simulink model "FocParamIdentifyModel"  (R2024a)
settings: Solver=FixedStepDiscrete  StartTime=0.0  StopTime=4  FixedStep=0.00005  RelTol=1e-3
values from neighbouring files (symbols this model uses):
  Flux = 0.00084    [FocParamIDFData.mat]
  Ld = 3.62e-05    [FocParamIDFData.mat]
  Lq = 4.24e-05    [FocParamIDFData.mat]
  Pole = 10    [FocParamIDFData.mat]
  Rs = 0.113    [FocParamIDFData.mat]
  Ts = 5e-05    [FocParamIDFData.mat]
undefined symbols (not defined in the file or in its folder): DiscIntNeverNeededParam, magnitude
libraries: slpidlib x4, mcbplantlib x1, autolibpmsmexterior x1
(part 1 of 2)
settings Model: Creator=张先生  LastModifiedBy=张先生
settings OptimizationCC: DefaultParameterBehavior=Inlined  UseDivisionForNetSlopeComputation=on  GainParamInheritBuiltInType=on  UseFloatMulNetSlope=on  InlineInvariantSignals=on  PassReuseOutputArgsAs=Individual arguments  ZeroExternalMemoryAtStartup=off  ZeroInternalMemoryAtStartup=off  NoFixptDivByZeroProtection=on  EfficientFloat2IntCast=on  LifeSpan=1  OptimizeBlockOrder=speed  DifferentSizesBufferReuse=on  EfficientTunableParamExpr=on
settings DebuggingCC: ParameterTunabilityLossMsg=error
settings HardwareCC: ProdBitPerPointer=32  ProdBitPerSizeT=32  ProdBitPerPtrDiffT=32  ProdLargestAtomicInteger=Long  ProdLargestAtomicFloat=Double  ProdWordSize=32  ProdLongLongMode=on  ProdHWDeviceType=ARM Compatible->ARM Cortex-M
settings SFSimCC: MATLABDynamicMemAlloc=off
settings RTWCC: Description=Embedded Coder  SystemTargetFile=ert.tlc  TemplateMakefile=ert_default_tmf  GenerateReport=on  LaunchReport=on
settings CodeAppCC: ForceParamTrailComments=on  IgnoreCustomStorageClasses=off  OperatorAnnotations=on  SimulinkDataObjDesc=on  SFDataObjDesc=on  CustomSymbolStrGlobalVar=rt$N$M  CustomSymbolStrType=$N$M  CustomSymbolStrFcn=$N$M$F  CustomSymbolStrMacro=$N$M  InsertBlockDesc=on
settings ERTTargetCC: TargetLangStandard=C99 (ISO)  CodeReplacementLibrary=ARM Cortex-M  GenerateSampleERTMain=on  IncludeMdlTerminateFcn=off  CombineSignalStateStructs=on  SupportComplex=off  SupportContinuousTime=on  SupportNonInlinedSFcns=on  InlinedParameterPlacement=NonHierarchical  ERTCustomFileTemplate=example_file_process.tlc  ERTFilePackagingFormat=CompactWithDataFile

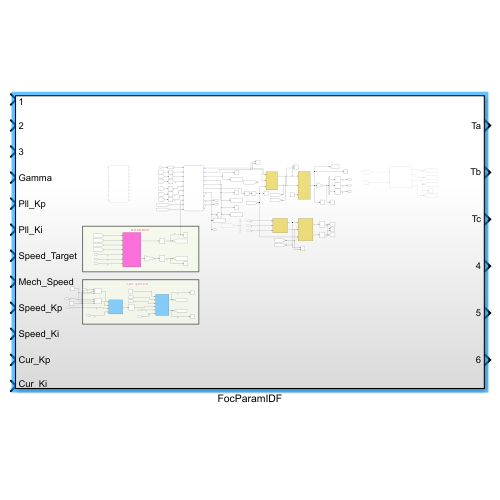
[thumbnail: Simulink's stored preview of the top-level diagram]
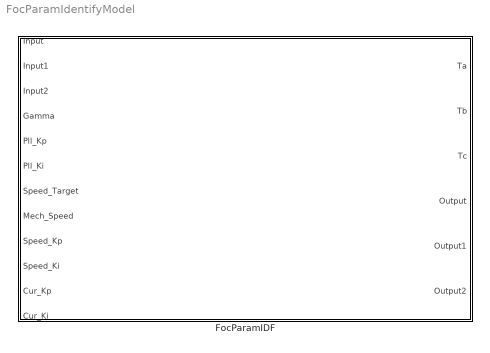
== system FocParamIdentifyModel ==
  FocParamIDF : Subsystem

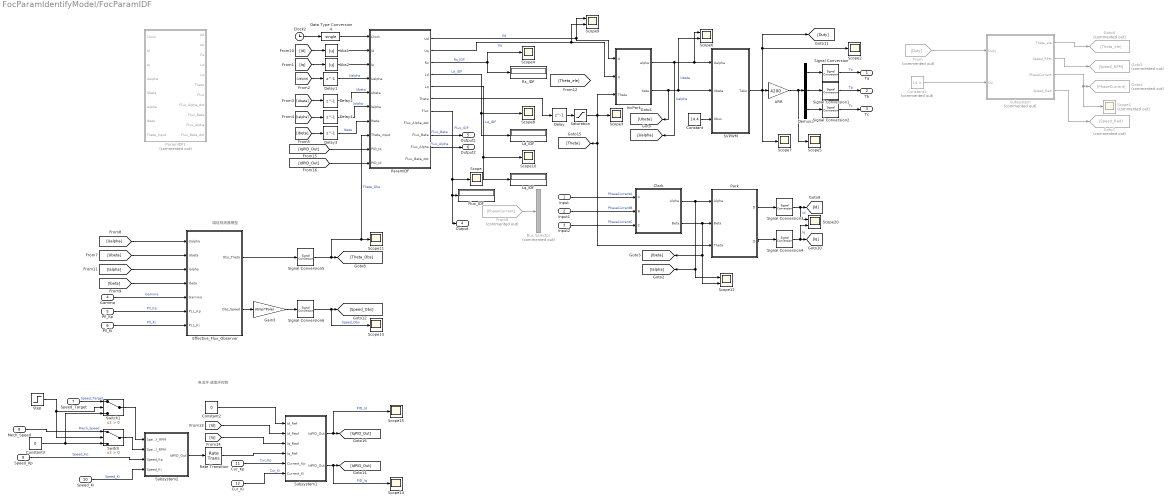
== system FocParamIdentifyModel/FocParamIDF ==
  note: 磁链观测器模型
  note: 电流环 速度环控制
  Input : Inport
  Input1 : Inport  Port=2
  Input2 : Inport  Port=3
  Gamma : Inport  Port=4
  Pll_Kp : Inport  Port=5
  Pll_Ki : Inport  Port=6
  Speed_Target : Inport  Port=7
  Mech_Speed : Inport  Port=8
  Speed_Kp : Inport  Port=9
  Speed_Ki : Inport  Port=10
  Cur_Kp : Inport  Port=11
  Cur_Ki : Inport  Port=12
  ARR : Gain  Gain=4200
  Abs1 : Abs  SaturateOnIntegerOverflow=off
  Abs2 : Abs  SaturateOnIntegerOverflow=off
  Bus Selector : BusSelector  Commented=on  OutputSignals=signal1,signal2,signal3
  Clark : Subsystem  TreatAsAtomicUnit=on
      settings: RTWSystemCode=Inline  RTWFcnNameOpts=Use subsystem name
      mask Display:
      | port_label('input',1,'a','texmode','on');
      | port_label('input',2,'b','texmode','on');
      | port_label('input',3,'c','texmode','on');
      | 
      | port_label('output',1,'\alpha','texmode','on');
      | port_label('output',2,'\beta','texmode','on');
      | 
      | fprintf('Clark');
  Clock2 : Clock
  Constant : Constant  Value=14.4  OutDataTypeStr=single
  Constant1 : Constant  Commented=on  Value=14.4  OutDataTypeStr=single
  Constant2 : Constant  Value=0  OutDataTypeStr=single
  Constant3 : Constant  Value=0  OutDataTypeStr=single
  Data Type Conversion4 : DataTypeConversion  OutDataTypeStr=single  SaturateOnIntegerOverflow=off  RndMeth=Floor
  Delay{,1..4} (5 alike) : Delay  DelayLength=1
  Demux3 : Demux  Outputs=3
  Effective_Flux_Observer : Subsystem
  Flux_IDF : Display
  From : From  Commented=on  GotoTag=Duty
  From6 : From  Commented=on  GotoTag=PhaseCurrent
  Gain3 : Gain  Gain=30/(pi*Pole)
  Goto4 : Goto  Commented=on  GotoTag=PhaseCurrent
  Goto5 : Goto  Commented=on  GotoTag=Speed_RPM
  Goto6 : Goto  Commented=on  GotoTag=Theta_ele
  Goto7 : Goto  Commented=on  GotoTag=Speed_Rad
  InvPark : Subsystem  TreatAsAtomicUnit=on
      settings: RTWFcnNameOpts=Use subsystem name
      mask Display:
      | port_label('input',1,'d','texmode','on');
      | port_label('input',2,'q','texmode','on');
      | port_label('input',3,'\theta','texmode','on');
      | 
      | port_label('output',1,'\alpha','texmode','on');
      | port_label('output',2,'\beta','texmode','on');
      | 
      | fprintf('Inverse\nPark')
  Ld_IDF : Display
  Lq_IDF : Display
  ParamIDF : Stateflow chart  TreatAsAtomicUnit=on
      settings: PortSchema="{\"entries\":[{\"content\":{\"sides\":[{\"content\":{\"connectorIds\":[\"In1\",\"In2\",\"In3\",\"In5\",\"In4\",\"In6\",\"In7\",\"In8\",\"In9\",\"In10\"]},\"type\":\"ConnectorPlacement.EquallySpacedRectSide\",\"uuid\":\"34403095-885b-4e18-8d39-de6823f4686e\"},{\"content\":{\"connectorIds\":[\"Out1\",\"Out3\",\"Out2\",\"Out4\",\"Out5\",\"Out6\",\"Out7\",\"Out8\",\"Out9\",\"Out10\",\"Out11\"],\"side\":\"RIGHT\"},\"type\":\"ConnectorPlacement.EquallySpacedRectSide\",\"uuid\":\"fe9f0ca0-7ade-4e8e-90a3-c920b6aed83b\"},{\"content\":{\"side\":\"TOP\"},\"type\":\"ConnectorPlacement.EquallySpacedRectSide\",\"uuid\":\"529ead30-0d9e-45e7-a0bb-7696b3472c65\"}]},\"type\":\"ConnectorPlacement.EquallySpacedConnector\",\"uuid\":\"00a1794a-fccb-4faf-9016-ac3359af7e1a\"}],\"packageUris\":[\"http://schema.mathworks.com/mf0/Connector/R2020b\"],\"version\":\"1.0\"}"
  ParamIDF1 : Stateflow chart  Commented=on  TreatAsAtomicUnit=on
      settings: PortSchema="{\"entries\":[{\"content\":{\"sides\":[{\"content\":{\"connectorIds\":[\"In1\",\"In2\",\"In3\",\"In5\",\"In4\",\"In6\",\"In7\",\"In8\"]},\"type\":\"ConnectorPlacement.EquallySpacedRectSide\",\"uuid\":\"34403095-885b-4e18-8d39-de6823f4686e\"},{\"content\":{\"connectorIds\":[\"Out1\",\"Out3\",\"Out2\",\"Out4\",\"Out5\",\"Out6\",\"Out7\",\"Out8\",\"Out9\",\"Out10\",\"Out11\"],\"side\":\"RIGHT\"},\"type\":\"ConnectorPlacement.EquallySpacedRectSide\",\"uuid\":\"fe9f0ca0-7ade-4e8e-90a3-c920b6aed83b\"},{\"content\":{\"side\":\"TOP\"},\"type\":\"ConnectorPlacement.EquallySpacedRectSide\",\"uuid\":\"529ead30-0d9e-45e7-a0bb-7696b3472c65\"}]},\"type\":\"ConnectorPlacement.EquallySpacedConnector\",\"uuid\":\"00a1794a-fccb-4faf-9016-ac3359af7e1a\"}],\"packageUris\":[\"http://schema.mathworks.com/mf0/Connector/R2020b\"],\"version\":\"1.0\"}"
  Park : Subsystem  TreatAsAtomicUnit=on
      settings: RTWFcnNameOpts=Use subsystem name
      mask Display:
      | port_label('input',1,'\alpha','texmode','on');
      | port_label('input',2, '\beta','texmode','on');
      | port_label('input',3, '\theta','texmode','on');
      | 
      | port_label('output',1,'d','texmode','on');
      | port_label('output',2,'q','texmode','on');
      | fprintf('Park');
  Rate Transition : RateTransition
  Rs_IDF : Display
  SVPWM : Subsystem  TreatAsAtomicUnit=on
  Saturation : Saturate  UpperLimit=2*pi-0.001  LowerLimit=-2*pi + 0.001
  Scope{,2..5,7..8,10..11,13..15} (12 alike) : Scope
  Scope1 : Scope  Commented=on
  Scope{6,9,12,20} (4 alike) : Scope  NumInputPorts=2
  Signal Conversion{,1..6} (7 alike) : SignalConversion  OverrideOpt=off
  Step : Step  Time=15  OutDataTypeStr=single  SampleTime=0
  Subsystem : Subsystem  Commented=on
  Subsystem1 : Subsystem
  Subsystem2 : Subsystem
  Switch : Switch  Criteria=u2 > Threshold  SaturateOnIntegerOverflow=off  InputSameDT=off
  Switch1 : Switch  Criteria=u2 > Threshold  SaturateOnIntegerOverflow=off  InputSameDT=off
  Ta : Outport
  Tb : Outport  Port=2
  Tc : Outport  Port=3
  Output : Outport  Port=4
  Output1 : Outport  Port=5
  Output2 : Outport  Port=6
  wires:
  Clark/2(Beta) -> Scope12/2, [Ibeta], Park/2(Beta)
  InvPark/1(alpha) -> Scope6/1, SVPWM/1(Ualpha), [Ualpha]  "Ualpha"
  InvPark/2(beta) -> Scope6/2, SVPWM/2(Ubeta), [Ubeta]  "Ubeta"
  Saturation/1 -> InvPark/3(Theta), Scope3/1, [Theta], Park/3(Theta)
  SVPWM/1(Tabc) -> Scope2/1, [Duty], ARR/1, Scope7/1
  ARR/1 -> Scope5/1, Demux3/1
  Park/1(D) -> Signal Conversion3/1
  Signal Conversion4/1 -> Scope20/2, [Iq]  "Iq"
  Signal Conversion2/1 -> Tc/1  "Tc"
  Signal Conversion3/1 -> Scope20/1, [Id]  "Id"
  Signal Conversion/1 -> Ta/1  "Ta"
  Demux3/2 -> Signal Conversion1/1
  Demux3/1 -> Signal Conversion/1
  Park/2(Q) -> Signal Conversion4/1
  Demux3/3 -> Signal Conversion2/1
  Clark/1(Alpha) -> Scope12/1, [Ialpha], Park/1(Alpha)
  Signal Conversion1/1 -> Tb/1  "Tb"
  Constant/1 -> SVPWM/3(Ubus)
  From/1 -> Subsystem/1(Duty)
  Constant1/1 -> Subsystem/2(DC)
  Subsystem/1(Theta_ele) -> Goto6/1
  Subsystem/2(Speed_RPM) -> Goto5/1
  Subsystem/3(PhaseCurrent) -> Scope1/1, Goto4/1
  From6/1 -> Bus Selector/1
  Clock2/1 -> Data Type Conversion4/1
  Data Type Conversion4/1 -> ParamIDF/1(Clock)
  ParamIDF/1(Ud) -> Scope9/1, InvPark/1(d)  "Ud"
  [Id] -> Abs1/1
  Abs1/1 -> ParamIDF/2(Id)
  ParamIDF/4(Ld) -> Scope8/1, Ld_IDF/1  "Ld_IDF"
  ParamIDF/5(Lq) -> Scope10/1, Lq_IDF/1  "Lq_IDF"
  ParamIDF/2(Rs) -> Scope4/1, Rs_IDF/1  "Rs_IDF"
  ParamIDF/3(Uq) -> Scope9/2, InvPark/2(q)  "Uq"
  [Iq] -> Abs2/1
  Abs2/1 -> ParamIDF/3(Iq)
  ParamIDF/6(Theta) -> Delay/1
  [Ualpha] -> Delay1/1
  [Ubeta] -> Delay2/1
  [Ialpha] -> Delay4/1
  [Ibeta] -> Delay3/1
  Delay1/1 -> ParamIDF/5(Ualpha)  "Ualpha"
  Delay2/1 -> ParamIDF/4(Ubeta)  "Ubeta"
  Delay3/1 -> ParamIDF/7(Ibeta)  "Ibeta"
  Delay4/1 -> ParamIDF/6(Ialpha)  "Ialpha"
  ParamIDF/7(Flux) -> Flux_IDF/1, Output/1, Scope/1  "Flux_IDF"
  Delay/1 -> Saturation/1
  Subsystem/4(Speed_Rad) -> Goto7/1
  Input/1 -> Clark/1(A)  "PhaseCurrentA"
  Input1/1 -> Clark/2(B)  "PhaseCurrentB"
  Input2/1 -> Clark/3(C)  "PhaseCurrentC"
  ParamIDF/9(Flux_Beta) -> Output1/1  "Flux_Beta"
  ParamIDF/10(Flux_Alpha) -> Output2/1  "Flux_Alpha"
  Effective_Flux_Observer/2(Obs_Speed) -> Gain3/1
  Signal Conversion5/1 -> [Theta_Obs], Scope11/1, ParamIDF/8(Theta_Input)  "Theta_Obs"
  Gain3/1 -> Signal Conversion6/1
  Pll_Ki/1 -> Effective_Flux_Observer/7(PLL_Ki)  "Pll_Ki"
  Signal Conversion6/1 -> Scope13/1, [Speed_Obs]  "Speed_Obs"
  Pll_Kp/1 -> Effective_Flux_Observer/6(PLL_Kp)  "Pll_Kp"
  Gamma/1 -> Effective_Flux_Observer/5(Gamma)  "Gamma"
  Effective_Flux_Observer/1(Obs_Theta) -> Signal Conversion5/1
  [Id] -> Subsystem1/2(Id_Real)
  Rate Transition/1 -> Subsystem1/4(Iq_Ref)
  Speed_Kp/1 -> Subsystem2/3(Speed_Kp)  "Speed_Kp"
  Cur_Ki/1 -> Subsystem1/6(Current_Ki)  "Cur_Ki"
  Constant2/1 -> Subsystem1/1(Id_Ref)
  Speed_Ki/1 -> Subsystem2/4(Speed_Ki)  "Speed_Ki"
  Subsystem1/1(IqPID_Out) -> Scope15/1, [IqPID_Out]  "PID_Id"
  [Iq] -> Subsystem1/3(Iq_Real)
  Subsystem1/2(IdPID_Out) -> Scope14/1, [IdPID_Out]  "PID_Iq"
  Cur_Kp/1 -> Subsystem1/5(Current_Kp)  "Cur_Kp"
  Subsystem2/1(IdPID_Out) -> Rate Transition/1
  [IqPID_Out] -> ParamIDF/9(PID_Iq)
  [IdPID_Out] -> ParamIDF/10(PID_Id)
  [Ualpha] -> Effective_Flux_Observer/1(Ualpha)
  [Ubeta] -> Effective_Flux_Observer/2(Ubeta)
  [Ialpha] -> Effective_Flux_Observer/3(Ialpha)
  [Ibeta] -> Effective_Flux_Observer/4(Ibeta)
  Mech_Speed/1 -> Switch/1  "Mech_Speed"
  Switch/1 -> Subsystem2/2(Speed_Real_RPM)
  Constant3/1 -> Switch1/3, Switch/3
  Step/1 -> Switch1/2, Switch/2
  Speed_Target/1 -> Switch1/1  "Speed_Target"
  Switch1/1 -> Subsystem2/1(Speed_Ref_RPM)

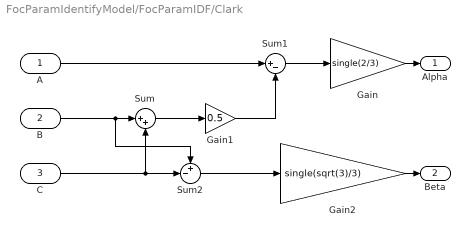
== system FocParamIdentifyModel/FocParamIDF/Clark ==
  A : Inport  OutDataTypeStr=single
  B : Inport  Port=2  OutDataTypeStr=single
  C : Inport  Port=3  OutDataTypeStr=single
  Gain : Gain  Gain=single(2/3)  OutDataTypeStr=single
  Gain1 : Gain  Gain=0.5  OutDataTypeStr=single
  Gain2 : Gain  Gain=single(sqrt(3)/3)  OutDataTypeStr=single
  Sum : Sum  Inputs=|++  OutDataTypeStr=single
  Sum1 : Sum  Inputs=|+-  OutDataTypeStr=single
  Sum2 : Sum  Inputs=+-|  OutDataTypeStr=single
  Alpha : Outport  OutDataTypeStr=single
  Beta : Outport  Port=2  OutDataTypeStr=single
  wires:
  Sum/1 -> Gain1/1
  Gain2/1 -> Beta/1
  B/1 -> Sum2/1, Sum/1
  Gain1/1 -> Sum1/2
  Gain/1 -> Alpha/1
  Sum2/1 -> Gain2/1
  C/1 -> Sum2/2, Sum/2
  A/1 -> Sum1/1
  Sum1/1 -> Gain/1

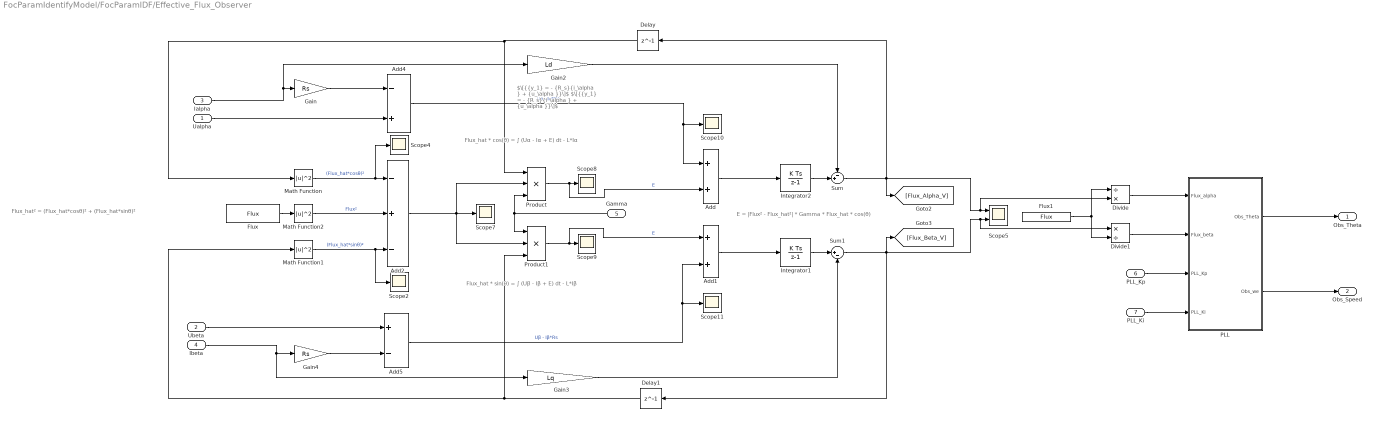
== system FocParamIdentifyModel/FocParamIDF/Effective_Flux_Observer ==
  note: Flux_hat² = (Flux_hat*cosθ)² + (Flux_hat*sinθ)²
  note: E = |Flux² - Flux_hat²| * Gamma * Flux_hat * cos(θ)
  note: Flux_hat * cos(θ) = ∫ (Uα - Iα + E) dt - L*Iα
  note: $\[{{y_1} = - {R_s}{i_\alpha } + {u_\alpha }}\]$ $\[{{y_1} = - {R_s}{i_\alpha } + {u_\alpha }}\]$
  note: Flux_hat * sin(θ) = ∫ (Uβ - Iβ + E) dt - L*Iβ
  Ualpha : Inport  OutDataTypeStr=single
  Ubeta : Inport  Port=2  OutDataTypeStr=single
  Ialpha : Inport  Port=3  OutDataTypeStr=single
  Ibeta : Inport  Port=4  OutDataTypeStr=single
  Gamma : Inport  Port=5
  PLL_Kp : Inport  Port=6
  PLL_Ki : Inport  Port=7
  Add : Sum  OutDataTypeStr=single
  Add1 : Sum  OutDataTypeStr=single
  Add2 : Sum  Inputs=-+-  OutDataTypeStr=single
  Add4 : Sum  Inputs=-+  OutDataTypeStr=single
  Add5 : Sum  Inputs=+-  OutDataTypeStr=single
  Delay : Delay  DelayLength=1
  Delay1 : Delay  DelayLength=1
  Divide : Product  Inputs=/*  OutDataTypeStr=single
  Divide1 : Product  Inputs=*/  OutDataTypeStr=single
  Flux : Constant  Value=Flux  OutDataTypeStr=double
  Flux1 : Constant  Value=Flux  OutDataTypeStr=double
  Gain : Gain  Gain=Rs  OutDataTypeStr=single
  Gain2 : Gain  Gain=Ld  OutDataTypeStr=single
  Gain3 : Gain  Gain=Lq  OutDataTypeStr=single
  Gain4 : Gain  Gain=Rs  OutDataTypeStr=single
  Integrator1 : DiscreteIntegrator  SampleTime=-1  OutDataTypeStr=single  ICPrevOutput=DiscIntNeverNeededParam  ICPrevScaledInput=DiscIntNeverNeededParam  mask(DiscretizedDiscreteIntegrator){}
      mask init:
      | %zoh
  Integrator2 : DiscreteIntegrator  SampleTime=-1  OutDataTypeStr=single  ICPrevOutput=DiscIntNeverNeededParam  ICPrevScaledInput=DiscIntNeverNeededParam  mask(DiscretizedDiscreteIntegrator){}
      mask init:
      | %zoh
  Math Function : Math  Operator=magnitude^2  OutDataTypeStr=single
  Math Function1 : Math  Operator=magnitude^2  OutDataTypeStr=single
  Math Function2 : Math  Operator=magnitude^2  OutDataTypeStr=single
  PLL : Subsystem
  Product : Product  Inputs=3  OutDataTypeStr=single
  Product1 : Product  Inputs=3  OutDataTypeStr=single
  Scope{2,4,7..11} (7 alike) : Scope
  Scope5 : Scope  NumInputPorts=2
  Sum : Sum  Inputs=-+|  OutDataTypeStr=single
  Sum1 : Sum  Inputs=|+-  OutDataTypeStr=single
  Obs_Theta : Outport
  Obs_Speed : Outport  Port=2
  wires:
  Gain2/1 -> Sum/1
  Gamma/1 -> Product1/1, Product/3
  Add5/1 -> Add1/2, Scope11/1  "Uβ - Iβ*Rs"
  Gain3/1 -> Sum1/2
  Integrator2/1 -> Sum/2
  Ialpha/1 -> Gain2/1, Gain/1
  Sum/1 -> [Flux_Alpha_V], Delay/1, Divide/2, Scope5/1
  Add4/1 -> Add/1, Scope10/1  "Uα - Iα*Rs"
  Add2/1 -> Scope7/1, Product1/2, Product/2
  Integrator1/1 -> Sum1/1
  Ibeta/1 -> Gain3/1, Gain4/1
  Sum1/1 -> Divide1/1, Scope5/2, [Flux_Beta_V], Delay1/1
  PLL/1(Obs_Theta) -> Obs_Theta/1
  Math Function1/1 -> Scope2/1, Add2/3  "(Flux_hat*sinθ)²"
  Math Function/1 -> Scope4/1, Add2/1  "(Flux_hat*cosθ)²"
  Product/1 -> Add/2, Scope8/1  "E"
  Product1/1 -> Add1/1, Scope9/1  "E"
  Flux/1 -> Math Function2/1
  Math Function2/1 -> Add2/2  "Flux²"
  Ubeta/1 -> Add5/1
  Gain4/1 -> Add5/2
  PLL/2(Obs_we) -> Obs_Speed/1
  Ualpha/1 -> Add4/2
  PLL_Kp/1 -> PLL/3(PLL_Kp)
  PLL_Ki/1 -> PLL/4(PLL_Ki)
  Add/1 -> Integrator2/1
  Add1/1 -> Integrator1/1
  Delay/1 -> Product/1, Math Function/1
  Delay1/1 -> Product1/3, Math Function1/1
  Gain/1 -> Add4/1
  Divide/1 -> PLL/1(Flux_alpha)
  Divide1/1 -> PLL/2(Flux_beta)
  Flux1/1 -> Divide1/2, Divide/1

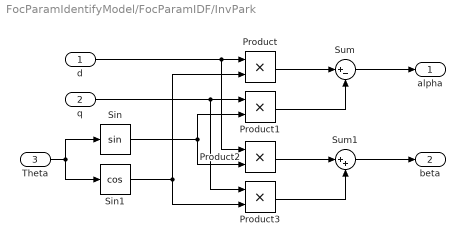
== system FocParamIdentifyModel/FocParamIDF/InvPark ==
  d : Inport  OutDataTypeStr=single
  q : Inport  Port=2  OutDataTypeStr=single
  Theta : Inport  Port=3  OutDataTypeStr=single
  Product{,1..3} (4 alike) : Product  OutDataTypeStr=single
  Sin : Trigonometry  ApproximationMethod=Lookup  TableDataTypeStr=single
  Sin1 : Trigonometry  Operator=cos  ApproximationMethod=Lookup  TableDataTypeStr=single
  Sum : Sum  Inputs=|+-  OutDataTypeStr=single
  Sum1 : Sum  Inputs=|++  OutDataTypeStr=single
  alpha : Outport  OutDataTypeStr=single
  beta : Outport  Port=2  OutDataTypeStr=single
  wires:
  Sum/1 -> alpha/1
  Theta/1 -> Sin1/1, Sin/1
  d/1 -> Product2/1, Product/1
  Sin1/1 -> Product/2, Product3/2
  q/1 -> Product3/1, Product1/1
  Sin/1 -> Product1/2, Product2/2
  Product/1 -> Sum/1
  Product1/1 -> Sum/2
  Product2/1 -> Sum1/1
  Product3/1 -> Sum1/2
  Sum1/1 -> beta/1

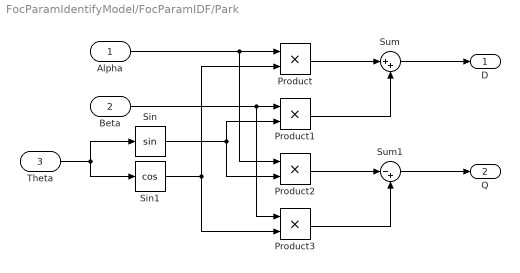
== system FocParamIdentifyModel/FocParamIDF/Park ==
  Alpha : Inport  OutDataTypeStr=single
  Beta : Inport  Port=2  OutDataTypeStr=single
  Theta : Inport  Port=3  OutDataTypeStr=single
  Product{,1..3} (4 alike) : Product  OutDataTypeStr=single
  Sin : Trigonometry  ApproximationMethod=Lookup  TableDataTypeStr=single
  Sin1 : Trigonometry  Operator=cos  ApproximationMethod=Lookup  TableDataTypeStr=single
  Sum : Sum  Inputs=|++  OutDataTypeStr=single
  Sum1 : Sum  Inputs=|-+  OutDataTypeStr=single
  D : Outport  OutDataTypeStr=single
  Q : Outport  Port=2  OutDataTypeStr=single
  wires:
  Beta/1 -> Product3/1, Product1/1
  Alpha/1 -> Product2/1, Product/1
  Theta/1 -> Sin1/1, Sin/1
  Sin1/1 -> Product/2, Product3/2
  Sin/1 -> Product1/2, Product2/2
  Product/1 -> Sum/1
  Product1/1 -> Sum/2
  Sum/1 -> D/1
  Product2/1 -> Sum1/1
  Product3/1 -> Sum1/2
  Sum1/1 -> Q/1

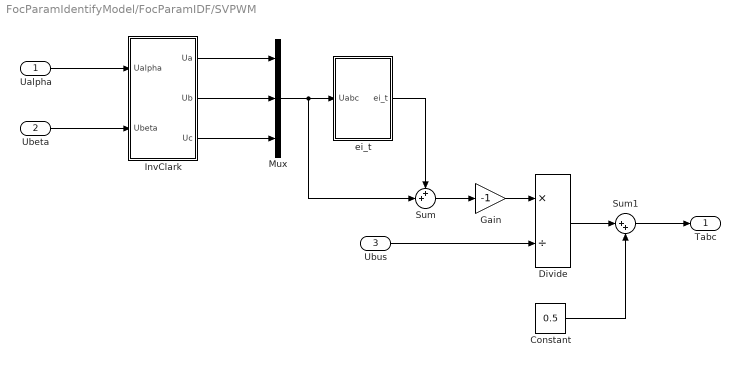
== system FocParamIdentifyModel/FocParamIDF/SVPWM ==
  Ualpha : Inport  OutDataTypeStr=single
  Ubeta : Inport  Port=2  OutDataTypeStr=single
  Ubus : Inport  Port=3  OutDataTypeStr=single
  Constant : Constant  Value=0.5  OutDataTypeStr=single
  Divide : Product  Inputs=*/  OutDataTypeStr=single
  Gain : Gain  Gain=-1  OutDataTypeStr=single
  InvClark : Subsystem
  Mux : Mux  Inputs=3
  Sum : Sum  Inputs=++|  OutDataTypeStr=single
  Sum1 : Sum  Inputs=|++  OutDataTypeStr=single
  ei_t : Subsystem
  Tabc : Outport  OutDataTypeStr=single
  wires:
  Ualpha/1 -> InvClark/1(Ualpha)
  Ubeta/1 -> InvClark/2(Ubeta)
  ei_t/1(ei_t) -> Sum/1
  InvClark/1(Ua) -> Mux/1
  InvClark/2(Ub) -> Mux/2
  InvClark/3(Uc) -> Mux/3
  Sum/1 -> Gain/1
  Mux/1 -> Sum/2, ei_t/1(Uabc)
  Divide/1 -> Sum1/1
  Constant/1 -> Sum1/2
  Ubus/1 -> Divide/2
  Gain/1 -> Divide/1
  Sum1/1 -> Tabc/1

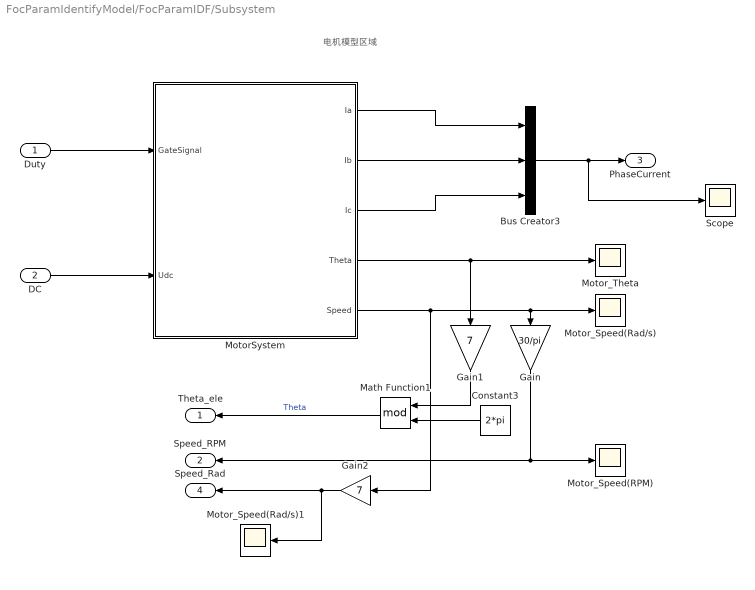
== system FocParamIdentifyModel/FocParamIDF/Subsystem ==
  note: 电机模型区域
  Duty : Inport
  DC : Inport  Port=2
  Bus Creator3 : BusCreator  Inputs=3
  Constant3 : Constant  Value=2*pi  OutDataTypeStr=single
  Gain : Gain  Gain=30/pi  OutDataTypeStr=single
  Gain1 : Gain  Gain=7  OutDataTypeStr=single
  Gain2 : Gain  Gain=7
  Math Function1 : Math  Operator=mod
  MotorSystem : Subsystem
  Motor_Speed(RPM) : Scope
  Motor_Speed(Rad/s) : Scope
  Motor_Speed(Rad/s)1 : Scope
  Motor_Theta : Scope
  Scope : Scope
  Theta_ele : Outport
  Speed_RPM : Outport  Port=2
  PhaseCurrent : Outport  Port=3
  Speed_Rad : Outport  Port=4
  wires:
  Duty/1 -> MotorSystem/1(GateSignal)
  MotorSystem/2(Ib) -> Bus Creator3/2
  Gain/1 -> Speed_RPM/1, Motor_Speed(RPM)/1
  MotorSystem/1(Ia) -> Bus Creator3/1
  MotorSystem/3(Ic) -> Bus Creator3/3
  Math Function1/1 -> Theta_ele/1  "Theta"
  MotorSystem/4(Theta) -> Motor_Theta/1, Gain1/1
  DC/1 -> MotorSystem/2(Udc)
  MotorSystem/5(Speed) -> Motor_Speed(Rad/s)/1, Gain/1, Gain2/1
  Constant3/1 -> Math Function1/2
  Gain1/1 -> Math Function1/1
  Bus Creator3/1 -> PhaseCurrent/1, Scope/1
  Gain2/1 -> Speed_Rad/1, Motor_Speed(Rad/s)1/1

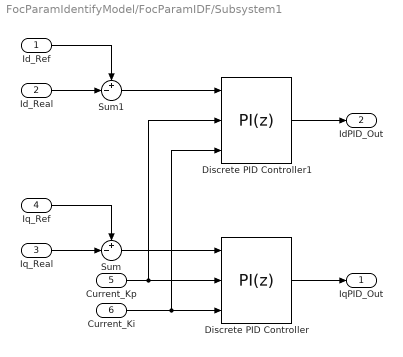
== system FocParamIdentifyModel/FocParamIDF/Subsystem1 ==
  Id_Ref : Inport
  Id_Real : Inport  Port=2
  Iq_Real : Inport  Port=3
  Iq_Ref : Inport  Port=4
  Current_Kp : Inport  Port=5
  Current_Ki : Inport  Port=6
  Discrete PID Controller : slpidlib/PID Controller  Controller=PI  Form=Parallel  TimeDomain=Discrete-time  UseExternalTs=off  SampleTime=-1  IntegratorMethod=Forward Euler  FilterMethod=Forward Euler  ControllerParametersSource=external  P=1  I=1  UseKiTs=off  D=0  UseExternalDerivativeSource=off  N=100  UseFilter=on  TunerSelectOption=Transfer Function Based (PID Tuner App)  InitialConditionSource=internal  InitialConditionForIntegrator=0  InitialConditionForFilter=0  DifferentiatorICPrevScaledInput=0  ExternalReset=none  TrackingMode=off  Kt=1  LimitOutput=on  SatLimitsSource=internal  UpperSaturationLimit=6.5  LowerSaturationLimit=-6.5  LinearizeAsGain=off  AntiWindupMode=clamping  Kb=1  LimitIntegrator=off  UpperIntegratorSaturationLimit=inf  LowerIntegratorSaturationLimit=-inf  SaturateOnIntegerOverflow=on  PGainOutDataTypeStr=single  PProdOutDataTypeStr=single  POutMin=[]  POutMax=[]  IGainOutDataTypeStr=single  IProdOutDataTypeStr=single  IOutMin=[]  IOutMax=[]  DOutMin=[]  DOutMax=[]  NOutMin=[]  NOutMax=[]  SumOutDataTypeStr=single  SumOutMin=[]  SumOutMax=[]  SaturationOutMin=[]  SaturationOutMax=[]  PParamMin=[]  PParamMax=[]  IParamMin=[]  IParamMax=[]  DParamMin=[]  DParamMax=[]  NParamMin=[]  NParamMax=[]  KbParamMin=[]  KbParamMax=[]  KtParamMin=[]  KtParamMax=[]  KbOutMin=[]  KbOutMax=[]  KtOutMin=[]  KtOutMax=[]  IntegratorOutMin=[]  IntegratorOutMax=[]  FilterOutMin=[]  FilterOutMax=[]  SumI1OutMin=[]  SumI1OutMax=[]  SumI2OutMin=[]  SumI2OutMax=[]  SumI3OutMin=[]  SumI3OutMax=[]  SumI4OutMin=[]  SumI4OutMax=[]  SumDOutMin=[]  SumDOutMax=[]  DifferentiatorOutMin=[]  DifferentiatorOutMax=[]  FilterDiffOutCoefMin=[]  FilterDiffOutCoefMax=[]  ReciprocalOutMin=[]  ReciprocalOutMax=[]  SumDenOutMin=[]  SumDenOutMax=[]  SumNumOutMin=[]  SumNumOutMax=[]  DivideOutMin=[]  DivideOutMax=[]  UdiffTsProdOutMin=[]  UdiffTsProdOutMax=[]  NTsProdOutMin=[]  NTsProdOutMax=[]  UintegralTsProdOutMin=[]  UintegralTsProdOutMax=[]  UngainTsProdOutMin=[]  UngainTsProdOutMax=[]  ClampingZeroOutDataTypeStr=Inherit: Inherit via back propagation  ClampingZeroOutMin=[]  ClampingZeroOutMax=[]  FilterDenConstantOutDataTypeStr=Inherit: Inherit via back propagation  FilterDenConstantOutMin=[]  FilterDenConstantOutMax=[]  PCopyOutDataTypeStr=Inherit: Inherit via back propagation  PCopyOutMin=[]  PCopyOutMax=[]  NCopyOutDataTypeStr=Inherit: Inherit via back propagation  NCopyOutMin=[]  NCopyOutMax=[]  IntegratorContinuousStateAttributes=''  IntegratorStateMustResolveToSignalObject=off  IntegratorRTWStateStorageClass=Auto  FilterContinuousStateAttributes=''  FilterStateMustResolveToSignalObject=off  FilterRTWStateStorageClass=Auto  ParallelPVariant=ExternalParameters  IdealPVariant=Disabled  IVariant=ExternalParameters  DVariant=Disabled  IntegratorVariant=Discrete  SatVariant=Enabled  AWVariant=DiscClampingParallel  PCopyVariant=Disabled  TRVariant=Disabled  FdbkBlocksVariant=Forward  IdealPFdbkVariant=Disabled  SatFdbkVariant=Disabled  DerivativeFilterVariant=Disabled  NVariant=Disabled  NCopyVariant=Disabled_SignalSpec  FilterICVariant=Disabled  IntegratorICVariant=InternalICs  ExternalResetVariant=Disabled  TRSumVariant=Passthrough  SumFdbkVariant=Disabled  SumVariant=Sum_PI  TsampFilterVariant=InternalTs  TsampNgainVariant=Passthrough  TsampIntegralVariant=Disabled_SignalSpec  ExternalSaturationOutDataTypeStr=Inherit: Same as second input  DerivativeSourceVariant=Disabled
      settings: LibrarySourceBlock=simulink/Discrete/Discrete PID Controller
  Discrete PID Controller1 : slpidlib/PID Controller  Controller=PI  Form=Parallel  TimeDomain=Discrete-time  UseExternalTs=off  SampleTime=-1  IntegratorMethod=Forward Euler  FilterMethod=Forward Euler  ControllerParametersSource=external  P=1  I=1  UseKiTs=off  D=0  UseExternalDerivativeSource=off  N=100  UseFilter=on  TunerSelectOption=Transfer Function Based (PID Tuner App)  InitialConditionSource=internal  InitialConditionForIntegrator=0  InitialConditionForFilter=0  DifferentiatorICPrevScaledInput=0  ExternalReset=none  TrackingMode=off  Kt=1  LimitOutput=on  SatLimitsSource=internal  UpperSaturationLimit=6.5  LowerSaturationLimit=-6.5  LinearizeAsGain=off  AntiWindupMode=clamping  Kb=1  LimitIntegrator=off  UpperIntegratorSaturationLimit=inf  LowerIntegratorSaturationLimit=-inf  SaturateOnIntegerOverflow=on  PGainOutDataTypeStr=single  PProdOutDataTypeStr=single  POutMin=[]  POutMax=[]  IGainOutDataTypeStr=single  IProdOutDataTypeStr=single  IOutMin=[]  IOutMax=[]  DOutMin=[]  DOutMax=[]  NOutMin=[]  NOutMax=[]  SumOutDataTypeStr=single  SumOutMin=[]  SumOutMax=[]  SaturationOutMin=[]  SaturationOutMax=[]  PParamMin=[]  PParamMax=[]  IParamMin=[]  IParamMax=[]  DParamMin=[]  DParamMax=[]  NParamMin=[]  NParamMax=[]  KbParamMin=[]  KbParamMax=[]  KtParamMin=[]  KtParamMax=[]  KbOutMin=[]  KbOutMax=[]  KtOutMin=[]  KtOutMax=[]  IntegratorOutMin=[]  IntegratorOutMax=[]  FilterOutMin=[]  FilterOutMax=[]  SumI1OutMin=[]  SumI1OutMax=[]  SumI2OutMin=[]  SumI2OutMax=[]  SumI3OutMin=[]  SumI3OutMax=[]  SumI4OutMin=[]  SumI4OutMax=[]  SumDOutMin=[]  SumDOutMax=[]  DifferentiatorOutMin=[]  DifferentiatorOutMax=[]  FilterDiffOutCoefMin=[]  FilterDiffOutCoefMax=[]  ReciprocalOutMin=[]  ReciprocalOutMax=[]  SumDenOutMin=[]  SumDenOutMax=[]  SumNumOutMin=[]  SumNumOutMax=[]  DivideOutMin=[]  DivideOutMax=[]  UdiffTsProdOutMin=[]  UdiffTsProdOutMax=[]  NTsProdOutMin=[]  NTsProdOutMax=[]  UintegralTsProdOutMin=[]  UintegralTsProdOutMax=[]  UngainTsProdOutMin=[]  UngainTsProdOutMax=[]  ClampingZeroOutDataTypeStr=Inherit: Inherit via back propagation  ClampingZeroOutMin=[]  ClampingZeroOutMax=[]  FilterDenConstantOutDataTypeStr=Inherit: Inherit via back propagation  FilterDenConstantOutMin=[]  FilterDenConstantOutMax=[]  PCopyOutDataTypeStr=Inherit: Inherit via back propagation  PCopyOutMin=[]  PCopyOutMax=[]  NCopyOutDataTypeStr=Inherit: Inherit via back propagation  NCopyOutMin=[]  NCopyOutMax=[]  IntegratorContinuousStateAttributes=''  IntegratorStateMustResolveToSignalObject=off  IntegratorRTWStateStorageClass=Auto  FilterContinuousStateAttributes=''  FilterStateMustResolveToSignalObject=off  FilterRTWStateStorageClass=Auto  ParallelPVariant=ExternalParameters  IdealPVariant=Disabled  IVariant=ExternalParameters  DVariant=Disabled  IntegratorVariant=Discrete  SatVariant=Enabled  AWVariant=DiscClampingParallel  PCopyVariant=Disabled  TRVariant=Disabled  FdbkBlocksVariant=Forward  IdealPFdbkVariant=Disabled  SatFdbkVariant=Disabled  DerivativeFilterVariant=Disabled  NVariant=Disabled  NCopyVariant=Disabled_SignalSpec  FilterICVariant=Disabled  IntegratorICVariant=InternalICs  ExternalResetVariant=Disabled  TRSumVariant=Passthrough  SumFdbkVariant=Disabled  SumVariant=Sum_PI  TsampFilterVariant=InternalTs  TsampNgainVariant=Passthrough  TsampIntegralVariant=Disabled_SignalSpec  ExternalSaturationOutDataTypeStr=Inherit: Same as second input  DerivativeSourceVariant=Disabled
      settings: LibrarySourceBlock=simulink/Discrete/Discrete PID Controller
  Sum : Sum  Inputs=+-|
  Sum1 : Sum  Inputs=+-|
  IqPID_Out : Outport
  IdPID_Out : Outport  Port=2
  wires:
  Sum/1 -> Discrete PID Controller/1
  Current_Kp/1 -> Discrete PID Controller/2, Discrete PID Controller1/2
  Iq_Ref/1 -> Sum/1
  Discrete PID Controller/1 -> IqPID_Out/1
  Current_Ki/1 -> Discrete PID Controller/3, Discrete PID Controller1/3
  Iq_Real/1 -> Sum/2
  Id_Ref/1 -> Sum1/1
  Id_Real/1 -> Sum1/2
  Sum1/1 -> Discrete PID Controller1/1
  Discrete PID Controller1/1 -> IdPID_Out/1

== system FocParamIdentifyModel/FocParamIDF/Subsystem2 ==
  Speed_Ref_RPM : Inport
  Speed_Real_RPM : Inport  Port=2
  Speed_Kp : Inport  Port=3
  Speed_Ki : Inport  Port=4
  Discrete PID Controller : slpidlib/PID Controller  Controller=PI  Form=Parallel  TimeDomain=Discrete-time  UseExternalTs=off  SampleTime=0.00025  IntegratorMethod=Forward Euler  FilterMethod=Forward Euler  ControllerParametersSource=external  P=1  I=1  UseKiTs=off  D=0  UseExternalDerivativeSource=off  N=100  UseFilter=on  TunerSelectOption=Transfer Function Based (PID Tuner App)  InitialConditionSource=internal  InitialConditionForIntegrator=0  InitialConditionForFilter=0  DifferentiatorICPrevScaledInput=0  ExternalReset=none  TrackingMode=off  Kt=1  LimitOutput=on  SatLimitsSource=internal  UpperSaturationLimit=20  LowerSaturationLimit=-20  LinearizeAsGain=off  AntiWindupMode=none  Kb=1  LimitIntegrator=off  UpperIntegratorSaturationLimit=inf  LowerIntegratorSaturationLimit=-inf  SaturateOnIntegerOverflow=on  PGainOutDataTypeStr=single  PProdOutDataTypeStr=single  POutMin=[]  POutMax=[]  IGainOutDataTypeStr=single  IProdOutDataTypeStr=single  IOutMin=[]  IOutMax=[]  DOutMin=[]  DOutMax=[]  NOutMin=[]  NOutMax=[]  SumOutDataTypeStr=single  SumOutMin=[]  SumOutMax=[]  SaturationOutMin=[]  SaturationOutMax=[]  PParamMin=[]  PParamMax=[]  IParamMin=[]  IParamMax=[]  DParamMin=[]  DParamMax=[]  NParamMin=[]  NParamMax=[]  KbParamMin=[]  KbParamMax=[]  KtParamMin=[]  KtParamMax=[]  KbOutMin=[]  KbOutMax=[]  KtOutMin=[]  KtOutMax=[]  IntegratorOutMin=[]  IntegratorOutMax=[]  FilterOutMin=[]  FilterOutMax=[]  SumI1OutMin=[]  SumI1OutMax=[]  SumI2OutMin=[]  SumI2OutMax=[]  SumI3OutMin=[]  SumI3OutMax=[]  SumI4OutMin=[]  SumI4OutMax=[]  SumDOutMin=[]  SumDOutMax=[]  DifferentiatorOutMin=[]  DifferentiatorOutMax=[]  FilterDiffOutCoefMin=[]  FilterDiffOutCoefMax=[]  ReciprocalOutMin=[]  ReciprocalOutMax=[]  SumDenOutMin=[]  SumDenOutMax=[]  SumNumOutMin=[]  SumNumOutMax=[]  DivideOutMin=[]  DivideOutMax=[]  UdiffTsProdOutMin=[]  UdiffTsProdOutMax=[]  NTsProdOutMin=[]  NTsProdOutMax=[]  UintegralTsProdOutMin=[]  UintegralTsProdOutMax=[]  UngainTsProdOutMin=[]  UngainTsProdOutMax=[]  ClampingZeroOutDataTypeStr=Inherit: Inherit via back propagation  ClampingZeroOutMin=[]  ClampingZeroOutMax=[]  FilterDenConstantOutDataTypeStr=Inherit: Inherit via back propagation  FilterDenConstantOutMin=[]  FilterDenConstantOutMax=[]  PCopyOutDataTypeStr=Inherit: Inherit via back propagation  PCopyOutMin=[]  PCopyOutMax=[]  NCopyOutDataTypeStr=Inherit: Inherit via back propagation  NCopyOutMin=[]  NCopyOutMax=[]  IntegratorContinuousStateAttributes=''  IntegratorStateMustResolveToSignalObject=off  IntegratorRTWStateStorageClass=Auto  FilterContinuousStateAttributes=''  FilterStateMustResolveToSignalObject=off  FilterRTWStateStorageClass=Auto  ParallelPVariant=ExternalParameters  IdealPVariant=Disabled  IVariant=ExternalParameters  DVariant=Disabled  IntegratorVariant=Discrete  SatVariant=Enabled  AWVariant=Passthrough  PCopyVariant=Disabled  TRVariant=Disabled  FdbkBlocksVariant=Forward  IdealPFdbkVariant=Disabled  SatFdbkVariant=Disabled  DerivativeFilterVariant=Disabled  NVariant=Disabled  NCopyVariant=Disabled_SignalSpec  FilterICVariant=Disabled  IntegratorICVariant=InternalICs  ExternalResetVariant=Disabled  TRSumVariant=Passthrough  SumFdbkVariant=Disabled  SumVariant=Sum_PI  TsampFilterVariant=InternalTs  TsampNgainVariant=Passthrough  TsampIntegralVariant=Disabled_SignalSpec  ExternalSaturationOutDataTypeStr=Inherit: Same as second input  DerivativeSourceVariant=Disabled
      settings: LibrarySourceBlock=simulink/Discrete/Discrete PID Controller
  Sum : Sum  Inputs=+-|
  IdPID_Out : Outport
  wires:
  Sum/1 -> Discrete PID Controller/1
  Speed_Kp/1 -> Discrete PID Controller/2
  Speed_Ref_RPM/1 -> Sum/1
  Discrete PID Controller/1 -> IdPID_Out/1
  Speed_Ki/1 -> Discrete PID Controller/3
  Speed_Real_RPM/1 -> Sum/2

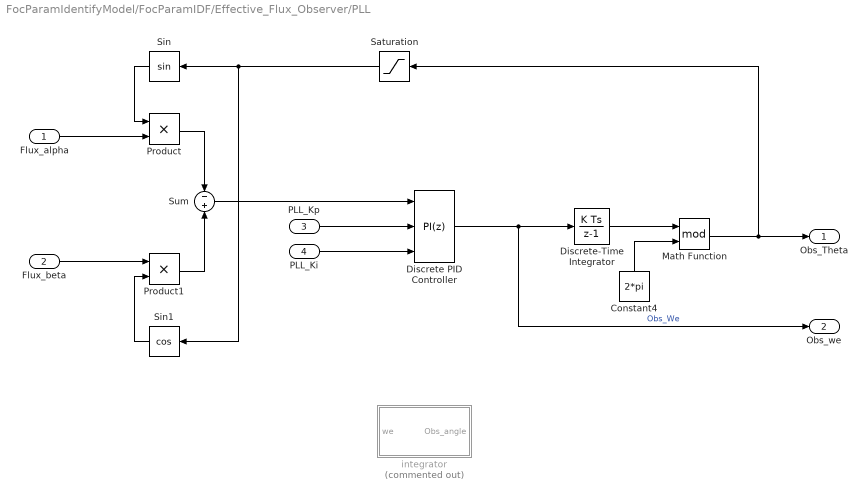
== system FocParamIdentifyModel/FocParamIDF/Effective_Flux_Observer/PLL ==
  Flux_alpha : Inport  OutDataTypeStr=single
  Flux_beta : Inport  Port=2  OutDataTypeStr=single
  PLL_Kp : Inport  Port=3
  PLL_Ki : Inport  Port=4
  Constant4 : Constant  Value=2*pi  OutDataTypeStr=single
  Discrete PID Controller : slpidlib/PID Controller  Controller=PI  Form=Parallel  TimeDomain=Discrete-time  UseExternalTs=off  SampleTime=-1  IntegratorMethod=Forward Euler  FilterMethod=Forward Euler  ControllerParametersSource=external  P=2*0.707*1650  I=1650*1650  UseKiTs=off  D=0  UseExternalDerivativeSource=off  N=100  UseFilter=on  TunerSelectOption=Transfer Function Based (PID Tuner App)  ZeroCross=off  InitialConditionSource=internal  InitialConditionForIntegrator=0  InitialConditionForFilter=0  DifferentiatorICPrevScaledInput=0  ExternalReset=none  TrackingMode=off  Kt=1  LimitOutput=on  SatLimitsSource=internal  UpperSaturationLimit=10566  LowerSaturationLimit=-10566  LinearizeAsGain=off  AntiWindupMode=clamping  Kb=1  LimitIntegrator=on  UpperIntegratorSaturationLimit=8797  LowerIntegratorSaturationLimit=-8797  SaturateOnIntegerOverflow=on  PGainOutDataTypeStr=single  PProdOutDataTypeStr=single  POutMin=[]  POutMax=[]  IGainOutDataTypeStr=single  IProdOutDataTypeStr=single  IOutMin=[]  IOutMax=[]  DOutMin=[]  DOutMax=[]  NOutMin=[]  NOutMax=[]  SumOutDataTypeStr=single  SumOutMin=[]  SumOutMax=[]  SaturationOutMin=[]  SaturationOutMax=[]  PParamMin=[]  PParamMax=[]  IParamMin=[]  IParamMax=[]  DParamMin=[]  DParamMax=[]  NParamMin=[]  NParamMax=[]  KbParamMin=[]  KbParamMax=[]  KtParamMin=[]  KtParamMax=[]  KbOutMin=[]  KbOutMax=[]  KtOutMin=[]  KtOutMax=[]  IntegratorOutMin=[]  IntegratorOutMax=[]  FilterOutMin=[]  FilterOutMax=[]  SumI1OutMin=[]  SumI1OutMax=[]  SumI2OutMin=[]  SumI2OutMax=[]  SumI3OutMin=[]  SumI3OutMax=[]  SumI4OutMin=[]  SumI4OutMax=[]  SumDOutMin=[]  SumDOutMax=[]  DifferentiatorOutMin=[]  DifferentiatorOutMax=[]  FilterDiffOutCoefMin=[]  FilterDiffOutCoefMax=[]  ReciprocalOutMin=[]  ReciprocalOutMax=[]  SumDenOutMin=[]  SumDenOutMax=[]  SumNumOutMin=[]  SumNumOutMax=[]  DivideOutMin=[]  DivideOutMax=[]  UdiffTsProdOutMin=[]  UdiffTsProdOutMax=[]  NTsProdOutMin=[]  NTsProdOutMax=[]  UintegralTsProdOutMin=[]  UintegralTsProdOutMax=[]  UngainTsProdOutMin=[]  UngainTsProdOutMax=[]  ClampingZeroOutDataTypeStr=Inherit: Inherit via back propagation  ClampingZeroOutMin=[]  ClampingZeroOutMax=[]  FilterDenConstantOutDataTypeStr=Inherit: Inherit via back propagation  FilterDenConstantOutMin=[]  FilterDenConstantOutMax=[]  PCopyOutDataTypeStr=Inherit: Inherit via back propagation  PCopyOutMin=[]  PCopyOutMax=[]  NCopyOutDataTypeStr=Inherit: Inherit via back propagation  NCopyOutMin=[]  NCopyOutMax=[]  IntegratorContinuousStateAttributes=''  IntegratorStateMustResolveToSignalObject=off  IntegratorRTWStateStorageClass=Auto  FilterContinuousStateAttributes=''  FilterStateMustResolveToSignalObject=off  FilterRTWStateStorageClass=Auto  ParallelPVariant=ExternalParameters  IdealPVariant=Disabled  IVariant=ExternalParameters  DVariant=Disabled  IntegratorVariant=Discrete  SatVariant=Enabled  AWVariant=DiscClampingParallel  PCopyVariant=Disabled  TRVariant=Disabled  FdbkBlocksVariant=Forward  IdealPFdbkVariant=Disabled  SatFdbkVariant=Disabled  DerivativeFilterVariant=Disabled  NVariant=Disabled  NCopyVariant=Disabled_SignalSpec  FilterICVariant=Disabled  IntegratorICVariant=InternalICs  ExternalResetVariant=Disabled  TRSumVariant=Passthrough  SumFdbkVariant=Disabled  SumVariant=Sum_PI  TsampFilterVariant=InternalTs  TsampNgainVariant=Passthrough  TsampIntegralVariant=Disabled_SignalSpec  ExternalSaturationOutDataTypeStr=Inherit: Same as second input  DerivativeSourceVariant=Disabled
  Discrete-Time Integrator : DiscreteIntegrator  SampleTime=-1  ICPrevOutput=DiscIntNeverNeededParam  ICPrevScaledInput=DiscIntNeverNeededParam
  Math Function : Math  Operator=mod
  Product : Product  OutDataTypeStr=single
  Product1 : Product  OutDataTypeStr=single
  Saturation : Saturate  UpperLimit=2*pi - 0.01  LowerLimit=-2*pi + 0.01
  Sin : Trigonometry  ApproximationMethod=Lookup
  Sin1 : Trigonometry  Operator=cos  ApproximationMethod=Lookup
  Sum : Sum  Inputs=-|+  OutDataTypeStr=single
  integrator : Subsystem  Commented=on
  Obs_Theta : Outport  OutDataTypeStr=single
  Obs_we : Outport  Port=2  OutDataTypeStr=single
  wires:
  Product/1 -> Sum/1
  Product1/1 -> Sum/2
  Sum/1 -> Discrete PID Controller/1
  Flux_alpha/1 -> Product/2
  Flux_beta/1 -> Product1/1
  Discrete PID Controller/1 -> Discrete-Time Integrator/1, Obs_we/1  "Obs_We"
  PLL_Ki/1 -> Discrete PID Controller/3
  PLL_Kp/1 -> Discrete PID Controller/2
  Sin/1 -> Product/1
  Sin1/1 -> Product1/2
  Math Function/1 -> Saturation/1, Obs_Theta/1
  Constant4/1 -> Math Function/2
  Discrete-Time Integrator/1 -> Math Function/1
  Saturation/1 -> Sin/1, Sin1/1

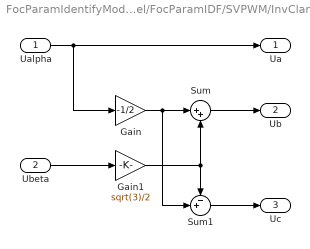
== system FocParamIdentifyModel/FocParamIDF/SVPWM/InvClark ==
  Ualpha : Inport  OutDataTypeStr=single
  Ubeta : Inport  Port=2  OutDataTypeStr=single
  Gain : Gain  Gain=-1/2  OutDataTypeStr=single
  Gain1 : Gain  Gain=sqrt(3)/2  OutDataTypeStr=single
  Sum : Sum  Inputs=|++  OutDataTypeStr=single
  Sum1 : Sum  Inputs=-+|  OutDataTypeStr=single
  Ua : Outport  OutDataTypeStr=single
  Ub : Outport  Port=2  OutDataTypeStr=single
  Uc : Outport  Port=3  OutDataTypeStr=single
  wires:
  Ualpha/1 -> Gain/1, Ua/1
  Ubeta/1 -> Gain1/1
  Gain/1 -> Sum1/2, Sum/1
  Sum/1 -> Ub/1
  Gain1/1 -> Sum/2, Sum1/1
  Sum1/1 -> Uc/1

== system FocParamIdentifyModel/FocParamIDF/SVPWM/ei_t ==
  Uabc : Inport  OutDataTypeStr=single
  Demux : Demux  Outputs=3
  Gain : Gain  Gain=-1/2  OutDataTypeStr=single
  Min : MinMax  Inputs=3  OutDataTypeStr=single
  Min1 : MinMax  Function=max  Inputs=3  OutDataTypeStr=single
  Sum : Sum  Inputs=|++  OutDataTypeStr=single
  ei_t : Outport  OutDataTypeStr=single
  wires:
  Min/1 -> Sum/1
  Sum/1 -> Gain/1
  Min1/1 -> Sum/2
  Gain/1 -> ei_t/1
  Uabc/1 -> Demux/1
  Demux/1 -> Min1/1, Min/1
  Demux/2 -> Min/2, Min1/2
  Demux/3 -> Min1/3, Min/3

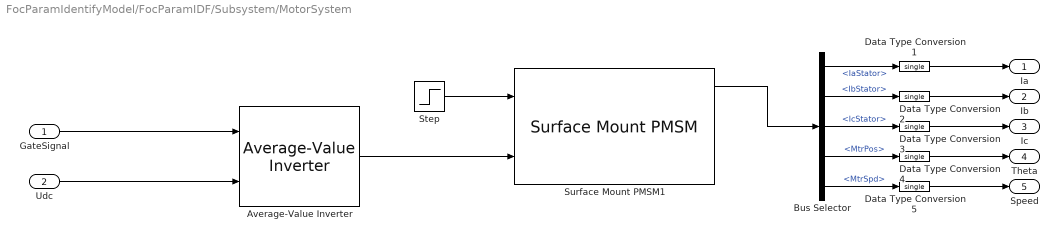
== system FocParamIdentifyModel/FocParamIDF/Subsystem/MotorSystem ==
  GateSignal : Inport
  Udc : Inport  Port=2
  Average-Value Inverter : mcbplantlib/Average-Value Inverter
  Bus Selector : BusSelector  OutputSignals=IaStator,IbStator,IcStator,MtrPos,MtrSpd
  Data Type Conversion{1..5} (5 alike) : DataTypeConversion  OutDataTypeStr=single  SaturateOnIntegerOverflow=off  RndMeth=Floor
  Step : Step  Time=1009  After=0  SampleTime=0.00005
  Surface Mount PMSM1 : autolibpmsmexterior/Surface Mount PMSM  port_config=Torque  sim_type=Discrete  Ts=0.00005  FilePath=E:\Sandbox\Bauto\Work\surfacepmsm_motordata.m  P=7  Rs=Rs  Ldq_=Ld  KConstText=Permanent flux linkage constant (lambda_pm):  lambda_pm=Flux  Ke=159.9771  Kt=1.323  mechanical=[1e-5, 1e-6, 0]  idq0=[0 0]  theta_init=0  omega_init=0  KConst=Flux  lambda_pm_calc=Flux  RefBlkName='autolibpmsmexterior/Surface Mount PMSM'  aMode=1  Ldq="[0.0003752   0.0003752]"
      settings: LibrarySourceBlock=autolibemachines/Surface Mount PMSM
  Ia : Outport
  Ib : Outport  Port=2
  Ic : Outport  Port=3
  Theta : Outport  Port=4
  Speed : Outport  Port=5
  wires:
  Bus Selector/5 -> Data Type Conversion5/1  "<MtrSpd>"
  Bus Selector/2 -> Data Type Conversion2/1  "<IbStator>"
  Bus Selector/3 -> Data Type Conversion3/1  "<IcStator>"
  Bus Selector/4 -> Data Type Conversion4/1  "<MtrPos>"
  Bus Selector/1 -> Data Type Conversion1/1  "<IaStator>"
  Average-Value Inverter/1 -> Surface Mount PMSM1/2
  Udc/1 -> Average-Value Inverter/2
  GateSignal/1 -> Average-Value Inverter/1
  Surface Mount PMSM1/1 -> Bus Selector/1
  Step/1 -> Surface Mount PMSM1/1
  Data Type Conversion1/1 -> Ia/1
  Data Type Conversion2/1 -> Ib/1
  Data Type Conversion3/1 -> Ic/1
  Data Type Conversion4/1 -> Theta/1
  Data Type Conversion5/1 -> Speed/1

== system FocParamIdentifyModel/FocParamIDF/Effective_Flux_Observer/PLL/integrator ==
  we : Inport  OutDataTypeStr=single
  Angle_Limit : Subsystem
  Delay : Delay  DelayLength=1
  Sum1 : Sum  Inputs=|++  OutDataTypeStr=single
  Ts : Gain  Gain=Ts  OutDataTypeStr=single
  Obs_angle : Outport  OutDataTypeStr=single
  wires:
  we/1 -> Ts/1
  Ts/1 -> Sum1/1
  Sum1/1 -> Angle_Limit/1(Angle_input)
  Delay/1 -> Obs_angle/1, Sum1/2
  Angle_Limit/1(Angle_output) -> Delay/1

== system FocParamIdentifyModel/FocParamIDF/Effective_Flux_Observer/PLL/integrator/Angle_Limit ==
  Angle_input : Inport
  If Action Subsystem1 : Subsystem  Commented=on  TreatAsAtomicUnit=on
  If Action Subsystem2 : Subsystem  Commented=on  TreatAsAtomicUnit=on
  If Action Subsystem3 : Subsystem  Commented=on  TreatAsAtomicUnit=on
  If1 : If  Commented=on  IfExpression=u1 > 6.283185307  ElseIfExpressions=u1<0
  MATLAB Function : MATLAB Function  TreatAsAtomicUnit=on
  Merge1 : Merge  Commented=on  Inputs=3
  Angle_output : Outport
  wires:
  If1/2 -> If Action Subsystem3/Action
  If1/1 -> If Action Subsystem2/Action
  If1/3 -> If Action Subsystem1/Action
  If Action Subsystem1/1(Out1) -> Merge1/3
  If Action Subsystem2/1(Out1) -> Merge1/1
  Angle_input/1 -> If Action Subsystem3/1(In1), If Action Subsystem1/1(In1), If Action Subsystem2/1(In1), MATLAB Function/1(in), If1/1
  If Action Subsystem3/1(Out1) -> Merge1/2
  MATLAB Function/1(out) -> Angle_output/1

== system FocParamIdentifyModel/FocParamIDF/Effective_Flux_Observer/PLL/integrator/Angle_Limit/If Action Subsystem1 ==
  In1 : Inport
  Action Port : ActionPort
  Out1 : Outport
  wires:
  In1/1 -> Out1/1

== system FocParamIdentifyModel/FocParamIDF/Effective_Flux_Observer/PLL/integrator/Angle_Limit/If Action Subsystem2 ==
  In1 : Inport
  Action Port : ActionPort
  2pi : Constant  Value=2*pi  OutDataTypeStr=single
  Subtract1 : Sum  Inputs=+-  OutDataTypeStr=single
  Out1 : Outport
  wires:
  In1/1 -> Subtract1/1
  Subtract1/1 -> Out1/1
  2pi/1 -> Subtract1/2

== system FocParamIdentifyModel/FocParamIDF/Effective_Flux_Observer/PLL/integrator/Angle_Limit/If Action Subsystem3 ==
  In1 : Inport
  Action Port : ActionPort
  Angle_offset : Constant  Value=2*pi  OutDataTypeStr=single
  Subtract1 : Sum
  Out1 : Outport
  wires:
  In1/1 -> Subtract1/1
  Subtract1/1 -> Out1/1
  Angle_offset/1 -> Subtract1/2

== matlab function FocParamIdentifyModel/FocParamIDF/Effective_Flux_Observer/PLL/integrator/Angle_Limit/MATLAB Function ==
  data: in input; out output
function out = fcn(in)
if in >= 2*pi
    out = in - 2*pi;
elseif in <= 0
    out = in + 2*pi;
else 
    out = in;
end

== stateflow chart FocParamIdentifyModel/FocParamIDF/ParamIDF ==
  state Ready
    en:
    Theta = single(0.0);
    Ud_t = single(0.0);
    Rs_t = single(0.0);
    Cnt = 1;
    Tim_Total = single(0.0);
    Uq = single(0.0);
    Ud = single(0.0);
    Ld = single(0.0);
    Lq = single(0.0);
    Ld_t = single(0.0);
    Lq_t = single(0.0);
  note: Ud缓慢增加阶段
  note: 计算电阻 累加阶段
  note: 平均电阻计算阶段
  note: 等待电流稳定
  state Rs_Stage1
    en:
    du:
    Ud_t = Ud_t + single(0.0001);
    Ud = Ud_t;
  state Rs_Stage4
    en:
    Ud = single(0.0);
    Uq = single(0.0);
    Cnt = 0;
    Tim_Total = single(0.0);
  state Rs_Stage2
    en:
    du:
    Rs_t = Rs_t + (Ud_t/Id)
    Cnt = Cnt + 1;
    Tim_Total = Tim_Total + single(0.00005);
  state Rs_Stage3
    en:
    Rs = Rs_t / single(1000.0)
  state Ld_Stage5
    en:
    Ud = single(0.0);
    Uq = single(0.0);
    Cnt = 0;
    Tim_Total = single(0.0);
  state Ld_State4
    en:
    Ld = Ld_t / single(Cnt);
    Cnt = 0;
  state Ld_State1
    en:
    Ud = single(1.0);
    Uq = single(0.0);
    du:
    Tim_Total = Tim_Total + single(0.00005);
  state Ld_State2
    en:
    Ud = single(0.0);
    Uq = single(0.0);
    Ld_t = Ld_t + (single(1.0)*Tim_Total)/Id;
    Cnt = Cnt + 1;
  state Ld_State3
    en:
    Ud = single(0.0);
    Uq = single(0.0);
    Tim_Total = single(0.0);
  state Lq_Stage5
    en:
    Ud = single(0.0);
    Uq = single(0.0);
    Cnt = 0;
    Tim_Total = single(0.0);
    du:
    Tim_Total = Tim_Total + single(0.00005);
  state Lq_State4
    en:
    Lq = Lq_t / single(Cnt);
    Cnt = 0;
  state Lq_State1
    en:
    Ud = single(0.0);
    Uq = single(1.0);
    du:
    Tim_Total = Tim_Total + single(0.00005);
  state Lq_State2
    en:
    Ud = single(0.0);
    Uq = single(0.0);
    Lq_t = Lq_t + (single(1.0)*Tim_Total/Iq);
    Cnt = Cnt + 1;
  state Lq_State3
    en:
    Ud = single(0.0);
    Uq = single(0.0);
    Tim_Total = single(0.0);
  note: 拖动电机以we = 20rad/s的速度旋转
  state Flux_State1
    en:
    Flux_Alpha_dot = single(0.0);
    Flux_Beta_dot = single(0.0);
    Flux_Alpha = single(0.0);
    Flux_Beta = single(0.0);
    Tim_Total = single(0.0);
    du:
    Flux_Alpha_dot = Ualpha - Rs*Ialpha;
    Flux_Beta_dot = Ubeta - Rs*Ibeta;
    Flux_Alpha = Flux_Alpha + Flux_Alpha_dot * single(0.00005);
    Flux_Beta = Flux_Beta + Flux_Beta_dot * single(0.00005);
    Flux = sqrt(Flux_Alpha*Flux_Alpha + Flux_Beta*Flux_Beta);
    if Theta < single(2*pi)
    Theta = Theta + single(0.0005);
    else
    Theta = single(0.0);
    end
    Tim_Total = Tim_Total + single(0.00005);
  state FluxObserver_Loop
    du:
    Ud = PID_Id;
    Uq = PID_Iq;
    Theta = Theta_Input;
    Tim_Total = single(0.0);
  state Flux_State0
    en:
    Tim_Total = single(0.0);
    Theta = 0;
    Uq = single(0.5);
    Ud = single(0.0);
    du:
    if Theta < single(2*pi)
    Theta = Theta + single(0.0005);
    else
    Theta = single(0.0);
    end
    Tim_Total = Tim_Total + single(0.00005);
  state Flux_State2
    en:
    Tim_Total = single(0.0);
    du:
    Ud = single(0.0);
    Uq = Uq - single(0.00005);
  note: Flux _Alpha_dot = Ualpha - Ialpha * Rs;
      | Flux_Beta_dot = Ubeta - Ibeta * Rs;
      | Flux = sqrt(Flux_Alpha² + Flux_Beta²);
  (default) -> Ready
  Rs_Stage1 -> Rs_Stage2 : [Id > 2]
  Ready -> Rs_Stage1 : [Clock > single(0.5)]
  Rs_Stage2 -> Rs_Stage3 : [Cnt > 1000]
  Rs_Stage3 -> Rs_Stage4
  Rs_Stage4 -> Ld_State1 : [Id <= single(0.001)&&Iq<= single(0.001)]
  Ld_State4 -> Ld_Stage5
  Ld_State1 -> Ld_State2 : [Tim_Total >= 0.0002]
  Ld_State3 -> Ld_State4 [order 2] : [Cnt >= 10]
  Ld_State2 -> Ld_State3
  Ld_Stage5 -> Lq_State1 : [Iq <= single(0.001) && Id <= single(0.001)]
  Ld_State3 -> Ld_State1 [order 1] : [Id < single(0.001)]
  Lq_State4 -> Lq_Stage5
  Lq_State3 -> Lq_State4 [order 2] : [Cnt >= 10]
  Lq_State2 -> Lq_State3
  Lq_State1 -> Lq_State2 : [Tim_Total >= 0.0002]
  Lq_Stage5 -> Flux_State0 : [Id <= single(0.001) && Iq <= single(0.001) && Tim_Total > single(0.5)]
  Lq_State3 -> Lq_State1 [order 1] : [Iq < single(0.001)]
  Flux_State0 -> Flux_State1 : [Tim_Total >= single(1.5)]
  Flux_State1 -> Flux_State2 : [Tim_Total > single(1.5)]
  Flux_State2 -> FluxObserver_Loop : [abs(Uq) <= single(0.01) && abs(Ud) <= single(0.01)]
  data: Ud output single; Ud_t local single; Rs_t local single; Cnt local int16; Clock input single; Rs output single; Id input single; Uq output single; Tim_Total local single; Iq input single; Ld output single; Lq output single; Ld_t local single; Lq_t local single; Theta output single; Ealpha local single; Ebeta local single; Ubeta input single; Ualpha input single; Ialpha input single; Ibeta input single; Flux output single; Flux_Alpha_dot output single; Flux_Beta output single; Flux_Alpha output single; Flux_Beta_dot output single; Theta_Input input single; PID_Iq input single; PID_Id input single
